simulink model "system_layout"  (R2021a)
settings: Solver=VariableStepAuto  StartTime=0.0  StopTime=20  RelTol=1e-3
model workspace (MAT data in the model file):
  m = 1
undefined symbols (not defined in the file): r
settings Model: Creator=Aiano  LastModifiedBy=Aiano

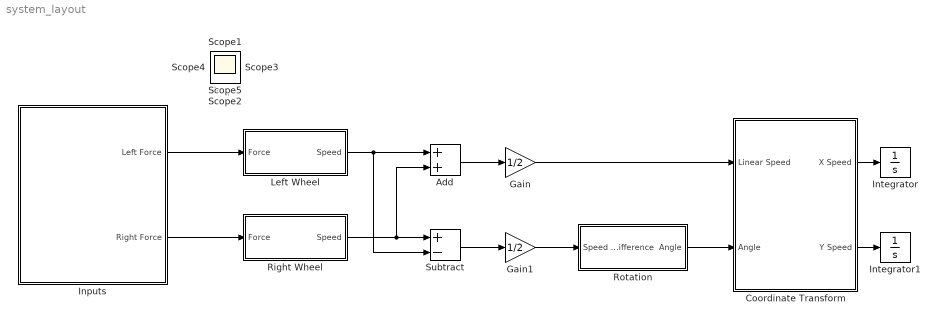
== system system_layout ==
  Add : Sum
  Coordinate Transform : Subsystem
  Gain : Gain  Gain=1/2
  Gain1 : Gain  Gain=1/2
  Inputs : Subsystem
  Integrator : Integrator
  Integrator1 : Integrator
  Left Wheel : Subsystem
  Right Wheel : Subsystem
  Rotation : Subsystem
  Subtract : Sum  Inputs=+-
  Scope{,1..5} (6 alike) : Scope
  wires:
  Right Wheel/1(Speed) -> Subtract/1, Add/2
  Add/1 -> Gain/1
  Subtract/1 -> Gain1/1
  Coordinate Transform/1(X Speed) -> Integrator/1
  Coordinate Transform/2(Y Speed) -> Integrator1/1
  Gain/1 -> Coordinate Transform/1(Linear Speed)
  Gain1/1 -> Rotation/1(Speed Difference)
  Rotation/1(Angle) -> Coordinate Transform/2(Angle)
  Inputs/2(Right Force) -> Right Wheel/1(Force)
  Inputs/1(Left Force) -> Left Wheel/1(Force)
  Left Wheel/1(Speed) -> Add/1, Subtract/2

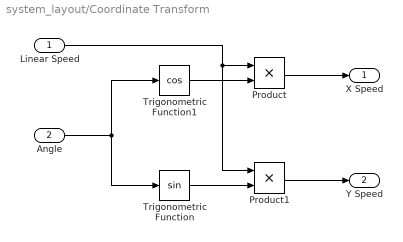
== system system_layout/Coordinate Transform ==
  Linear Speed : Inport
  Angle : Inport  Port=2
  Product : Product
  Product1 : Product
  Trigonometric Function : Trigonometry
  Trigonometric Function1 : Trigonometry  Operator=cos
  X Speed : Outport
  Y Speed : Outport  Port=2
  wires:
  Angle/1 -> Trigonometric Function/1, Trigonometric Function1/1
  Trigonometric Function1/1 -> Product/2
  Linear Speed/1 -> Product/1, Product1/1
  Trigonometric Function/1 -> Product1/2
  Product/1 -> X Speed/1
  Product1/1 -> Y Speed/1

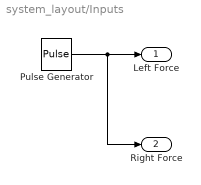
== system system_layout/Inputs ==
  Pulse Generator : DiscretePulseGenerator  PulseType=Time based  Period=20  PulseWidth=15
  Left Force : Outport
  Right Force : Outport  Port=2
  wires:
  Pulse Generator/1 -> Left Force/1, Right Force/1

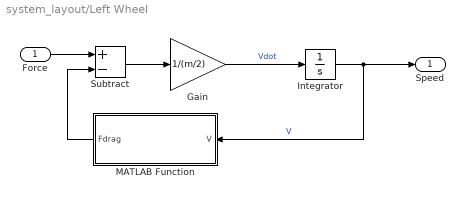
== system system_layout/Left Wheel ==
  Force : Inport
  Gain : Gain  Gain=1/(m/2)
  Integrator : Integrator
  MATLAB Function : MATLAB Function  TreatAsAtomicUnit=on
  Subtract : Sum  Inputs=+-
  Speed : Outport
  wires:
  Subtract/1 -> Gain/1
  Force/1 -> Subtract/1
  Integrator/1 -> MATLAB Function/1(V), Speed/1  "V"
  MATLAB Function/1(Fdrag) -> Subtract/2
  Gain/1 -> Integrator/1  "Vdot"

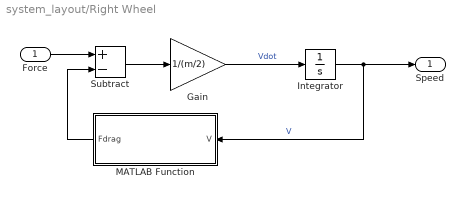
== system system_layout/Right Wheel ==
  Force : Inport
  Gain : Gain  Gain=1/(m/2)
  Integrator : Integrator
  MATLAB Function : MATLAB Function  TreatAsAtomicUnit=on
  Subtract : Sum  Inputs=+-
  Speed : Outport
  wires:
  Force/1 -> Subtract/1
  MATLAB Function/1(Fdrag) -> Subtract/2
  Subtract/1 -> Gain/1
  Gain/1 -> Integrator/1  "Vdot"
  Integrator/1 -> MATLAB Function/1(V), Speed/1  "V"

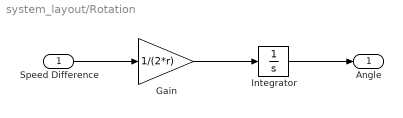
== system system_layout/Rotation ==
  Speed Difference : Inport
  Gain : Gain  Gain=1/(2*r)
  Integrator : Integrator
  Angle : Outport
  wires:
  Speed Difference/1 -> Gain/1
  Gain/1 -> Integrator/1
  Integrator/1 -> Angle/1

== matlab function system_layout/Right Wheel/MATLAB Function ==
  data: V input; Fdrag output; k_drag parameter
function Fdrag  = get_fdrag(V, k_drag)

Fdrag = k_drag*V*abs(V);

== matlab function system_layout/Left Wheel/MATLAB Function ==
  data: V input; Fdrag output; k_drag parameter
function Fdrag  = get_fdrag(V, k_drag)

Fdrag = k_drag*V*abs(V);
